simulink model "equation"  (R2019a)
settings: Solver=ode3  StartTime=0.0  StopTime=100.0  FixedStep=0.01  RelTol=1e-3
undefined symbols (not defined in the file): a, b, d, w
settings Model: Creator=lab  LastModifiedBy=lab
settings DataIOCC: SaveFormat=Array  ReturnWorkspaceOutputs=off

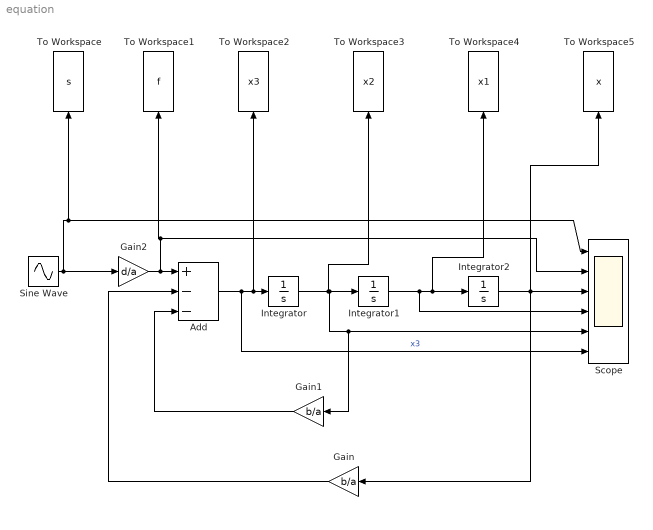
== system equation ==
  Add : Sum  Inputs=+--
  Gain : Gain  Gain=b/a
  Gain1 : Gain  Gain=b/a
  Gain2 : Gain  Gain=d/a
  Integrator : Integrator  InitialCondition=-0.02
  Integrator1 : Integrator  InitialCondition=-0.02
  Integrator2 : Integrator  InitialCondition=w
  Scope : Scope  NumInputPorts=6
  Sine Wave : Sin  Amplitude=4  Frequency=12  SampleTime=0
  To Workspace : ToWorkspace  VariableName=s  SampleTime=-1
  To Workspace1 : ToWorkspace  VariableName=f  SampleTime=-1
  To Workspace2 : ToWorkspace  VariableName=x3  SampleTime=-1
  To Workspace3 : ToWorkspace  VariableName=x2  SampleTime=-1
  To Workspace4 : ToWorkspace  VariableName=x1  SampleTime=-1
  To Workspace5 : ToWorkspace  VariableName=x  SampleTime=-1
  wires:
  Integrator/1 -> To Workspace3/1, Gain1/1, Scope/5, Integrator1/1
  Integrator1/1 -> Scope/4, To Workspace4/1, Integrator2/1
  Integrator2/1 -> To Workspace5/1, Scope/3, Gain/1
  Add/1 -> Scope/6, To Workspace2/1, Integrator/1  "x3"
  Gain2/1 -> Scope/2, To Workspace1/1, Add/1
  Sine Wave/1 -> Scope/1, To Workspace/1, Gain2/1
  Gain/1 -> Add/2
  Gain1/1 -> Add/3
